simulink model "Problem5_Circuit_Simulation"  (R2020b)
settings: Solver=VariableStepAuto  StartTime=0.0  StopTime=10  RelTol=1e-3
values from neighbouring files (symbols this model uses):
  C = 1e-05    [Data.mat]
  R = 10    [Data.mat]
settings Model: Creator=vigne  LastModifiedBy=vigne

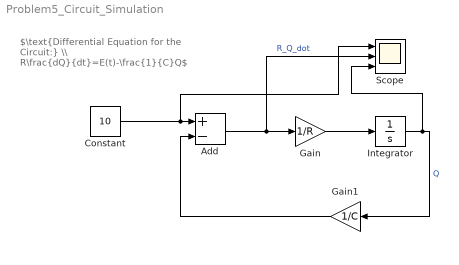
== system Problem5_Circuit_Simulation ==
  note: $\text{Differential Equation for the Circuit:} \\ R\frac{dQ}{dt}=E(t)-\frac{1}{C}Q$
  Add : Sum  Inputs=+-
  Constant : Constant  Value=10
  Gain : Gain  Gain=1/R
  Gain1 : Gain  Gain=1/C
  Integrator : Integrator  InitialCondition=5
  Scope : Scope  NumInputPorts=3
  wires:
  Add/1 -> Scope/2, Gain/1  "R_Q_dot"
  Gain/1 -> Integrator/1
  Integrator/1 -> Scope/3, Gain1/1  "Q"
  Gain1/1 -> Add/2
  Constant/1 -> Scope/1, Add/1
